simulink model "bio_matfunc_DCM_to_quat"  (R2017b)
settings: Solver=VariableStepAuto  StartTime=0.0  StopTime=10.0  RelTol=1e-3
settings Model: Creator=ktrinh  LastModifiedBy=ktrinh

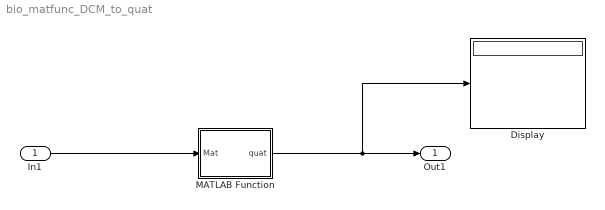
== system bio_matfunc_DCM_to_quat ==
  In1 : Inport  OutDataTypeStr=double  PortDimensions=[3,3]
  Display : Display
  MATLAB Function : MATLAB Function  TreatAsAtomicUnit=on
  Out1 : Outport
  wires:
  MATLAB Function/1(quat) -> Display/1, Out1/1
  In1/1 -> MATLAB Function/1(Mat)

== matlab function bio_matfunc_DCM_to_quat/MATLAB Function ==
  data: Mat input; quat output
function quat = DCM_to_quat(Mat)
%#codegen
Mat = Mat';

Mxx = Mat(1,1);
Myy = Mat(2,2);
Mzz = Mat(3,3);
Mxy = Mat(1,2);
Myx = Mat(2,1);
Mxz = Mat(1,3);
Mzx = Mat(3,1);
Myz = Mat(2,3);
Mzy = Mat(3,2);

a =  Mxx + Myy + Mzz;
b =  Mxx - Myy - Mzz;
c = -Mxx + Myy - Mzz;
d = -Mxx - Myy + Mzz;


if a > 0
    e = 2*sqrt(1+a);
    Qx = (Mzy - Myz)/e;
    Qy = (Mxz - Mzx)/e;
    Qz = (Myx - Mxy)/e;
    Qs = e/4;
    
elseif (Mxx > Myy) && (Mxx > Mzz)
    e = 2*sqrt(1 + b);
    Qx = e/4;
    Qy = (Mxy + Myx)/e;
    Qz = (Mxz + Mzx)/e;
    Qs = (Mzy - Myz)/e;
    
elseif Myy > Mzz
    e = 2*sqrt(1 + c);
    Qx = (Mxy + Myx)/e;
    Qy = e/4;
    Qz = (Myz + Mzy)/e;
    Qs = (Mxz - Mzx)/e;
    
else
    e = 2*sqrt(1 + d);
    Qx = (Mxz + Mzx)/e;
    Qy = (Myz + Mzy)/e;
    Qz = e/4;
    Qs = (Myx - Mxy)/e;
    
end

quatMag = sqrt(Qx^2 + Qy^2 + Qz^2 + Qs^2);

quat = [Qx/quatMag, Qy/quatMag, Qz/quatMag, Qs/quatMag]';
